simulink model "top_model_rw_desatTest"  (R2017b)
settings: Solver=FixedStepAuto  StartTime=0.0  StopTime=30000  FixedStep=.2  RelTol=1e-3  EnableMultiTasking=on
model workspace: external: MATLAB File C:\Users\Justin\Documents\00 MEng Project\PAN_ADCS\initialization\simulink_workspace_init.m (data not in the file)
undefined symbols (not defined in the file): h_init, hdmax, hmax, IAU, Imp_max, Imp_min, init, K_F, Kd, km, Kp, L_F, m_follower, match_tol, muE, ontime_max, ontime_min, q_init, s, Thrust_max, Thrust_min, wbn_init
libraries: aerolibtransform2 x12, aerolibconvert2 x8, sharedtransform x8, hEemethod x8, aerolibgravity2 x6, aerolibutil x6, aerolibcelestial x4, vrlib x4
(part 1 of 5)
settings Model: Creator=The MathWorks, Inc.  LastModifiedBy=Justin
settings DataIOCC: LimitDataPoints=on
settings OptimizationCC: LifeSpan=inf
settings DebuggingCC: AllowSymbolicDim=off  SFUnexpectedBacktrackingDiag=warning  SFNoUnconditionalDefaultTransitionDiag=warning  SFExecutionAtInitializationDiag=none
settings ModelReferenceCC: PropagateSignalLabelsOutOfModel=off
settings CodeAppCC: StateflowObjectComments=on
settings GRTTargetCC: TargetLangStandard=C89/C90 (ANSI)
settings ConfigComp: CovMetricSettings=dw  CovHtmlReporting=on  CovSaveCumulativeToWorkspaceVar=on  CovSaveSingleToWorkspaceVar=on  CovExternalEMLEnable=off

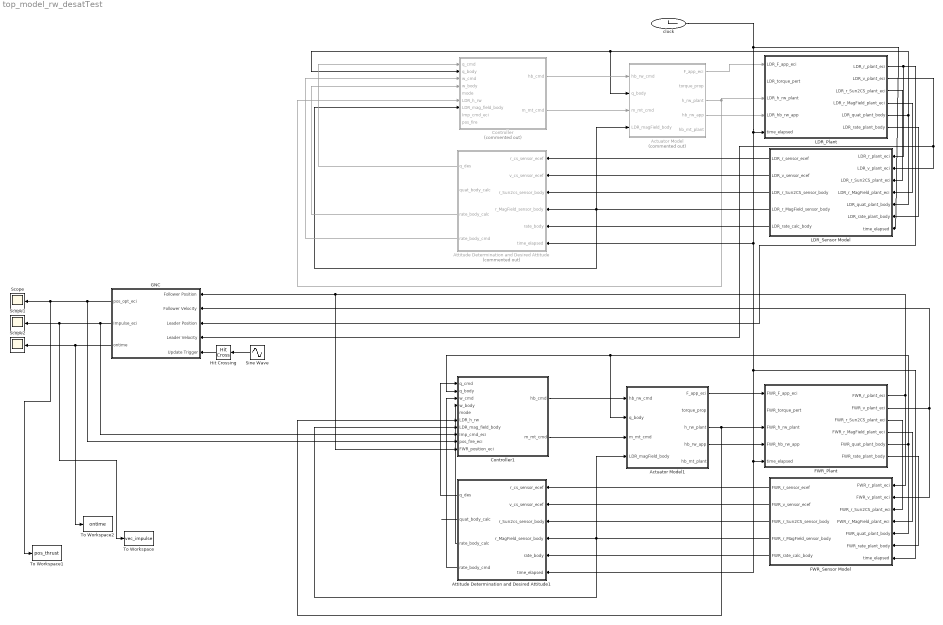
== system top_model_rw_desatTest ==
  Actuator Model : Subsystem  Commented=on
  Actuator Model1 : Subsystem
  Attitude Determination and Desired Attitude : Subsystem  Commented=on
  Attitude Determination and Desired Attitude1 : Subsystem
  Controller : Subsystem  Commented=on
  Controller1 : Subsystem
  FWR_Plant : Subsystem
  FWR_Sensor Model : Subsystem
  GNC : Subsystem
  Hit Crossing : HitCross  HitCrossingOffset=0.5  HitCrossingDirection=rising
  LDR_Plant : Subsystem
  LDR_Sensor Model : Subsystem
  Scope : Scope
  Scope1 : Scope
  Scope2 : Scope
  Sine Wave : Sin  Frequency=2*pi/550  SampleTime=0
  To Workspace : ToWorkspace  VariableName=vec_impulse  SaveFormat=Timeseries  SampleTime=-1
  To Workspace1 : ToWorkspace  VariableName=pos_thrust  SaveFormat=Timeseries  SampleTime=-1
  To Workspace2 : ToWorkspace  VariableName=ontime  SaveFormat=Timeseries  SampleTime=-1
  clock : Clock
      settings: Decimation=100
  wires:
  LDR_Plant/3(LDR_r_Sun2CS_plant_eci) -> LDR_Sensor Model/3(LDR_r_Sun2CS_plant_eci)
  LDR_Plant/4(LDR_r_MagField_plant_eci) -> LDR_Sensor Model/4(LDR_r_MagField_plant_eci)
  LDR_Plant/6(LDR_rate_plant_body) -> LDR_Sensor Model/6(LDR_rate_plant_body)
  Actuator Model/1(F_app_eci) -> LDR_Plant/1(LDR_F_app_eci)
  Actuator Model/3(h_rw_plant) -> Controller/6(LDR_h_rw), LDR_Plant/3(LDR_h_rw_plant)
  Actuator Model/4(hb_rw_app) -> LDR_Plant/4(LDR_hb_rw_app)
  LDR_Sensor Model/1(LDR_r_sensor_ecef) -> Attitude Determination and Desired Attitude/1(r_cs_sensor_ecef)
  LDR_Sensor Model/2(LDR_v_sensor_ecef) -> Attitude Determination and Desired Attitude/2(v_cs_sensor_ecef)
  LDR_Sensor Model/3(LDR_r_Sun2CS_sensor_body) -> Attitude Determination and Desired Attitude/3(r_Sun2cs_sensor_body)
  LDR_Sensor Model/4(LDR_r_MagField_sensor_body) -> Controller/7(LDR_mag_field_body), Attitude Determination and Desired Attitude/4(r_MagField_sensor_body), Actuator Model/4(LDR_magField_body)
  LDR_Sensor Model/5(LDR_rate_calc_body) -> Attitude Determination and Desired Attitude/5(rate_body)
  GNC/1(pos_opt_eci) -> Controller1/9(pos_fire_eci), To Workspace1/1, Scope/1
  GNC/2(Impulse_eci) -> Controller1/8(Imp_cmd_eci), To Workspace/1, Scope1/1
  GNC/3(ontime) -> To Workspace2/1, Scope2/1
  Sine Wave/1 -> Hit Crossing/1
  Hit Crossing/1 -> GNC/5(Update Trigger)
  LDR_Plant/5(LDR_quat_plant_body) -> LDR_Sensor Model/5(LDR_quat_plant_body), Actuator Model/2(q_body), Controller/2(q_body)
  Attitude Determination and Desired Attitude/1(q_des) -> Controller/1(q_cmd)
  Attitude Determination and Desired Attitude/3(rate_body_calc) -> Controller/4(w_body)
  Controller/1(hb_cmd) -> Actuator Model/1(hb_rw_cmd)
  Controller/2(m_mt_cmd) -> Actuator Model/3(m_mt_cmd)
  Attitude Determination and Desired Attitude/4(rate_body_cmd) -> Controller/3(w_cmd)
  LDR_Plant/1(LDR_r_plant_eci) -> GNC/3(Leader Position), LDR_Sensor Model/1(LDR_r_plant_eci)
  LDR_Plant/2(LDR_v_plant_eci) -> GNC/4(Leader Velocity), LDR_Sensor Model/2(LDR_v_plant_eci)
  FWR_Plant/2(FWR_v_plant_eci) -> FWR_Sensor Model/2(FWR_v_plant_eci), GNC/2(Follower Velocity)
  FWR_Plant/5(FWR_quat_plant_body) -> FWR_Sensor Model/5(FWR_quat_plant_body), Actuator Model1/2(q_body), Controller1/2(q_body)
  Controller1/2(m_mt_cmd) -> Actuator Model1/3(m_mt_cmd)
  FWR_Sensor Model/3(FWR_r_Sun2CS_sensor_body) -> Attitude Determination and Desired Attitude1/3(r_Sun2cs_sensor_body)
  FWR_Sensor Model/2(FWR_v_sensor_ecef) -> Attitude Determination and Desired Attitude1/2(v_cs_sensor_ecef)
  FWR_Sensor Model/1(FWR_r_sensor_ecef) -> Attitude Determination and Desired Attitude1/1(r_cs_sensor_ecef)
  Controller1/1(hb_cmd) -> Actuator Model1/1(hb_rw_cmd)
  FWR_Plant/3(FWR_r_Sun2CS_plant_eci) -> FWR_Sensor Model/3(FWR_r_Sun2CS_plant_eci)
  FWR_Plant/6(FWR_rate_plant_body) -> FWR_Sensor Model/6(FWR_rate_plant_body)
  FWR_Sensor Model/4(FWR_r_MagField_sensor_body) -> Controller1/7(LDR_mag_field_body), Attitude Determination and Desired Attitude1/4(r_MagField_sensor_body), Actuator Model1/4(LDR_magField_body)
  Actuator Model1/3(h_rw_plant) -> Controller1/6(LDR_h_rw), FWR_Plant/3(FWR_h_rw_plant)
  clock/1 -> LDR_Sensor Model/7(time_elapsed), FWR_Sensor Model/7(time_elapsed), Attitude Determination and Desired Attitude1/6(time_elapsed), FWR_Plant/5(time_elapsed), Attitude Determination and Desired Attitude/6(time_elapsed), LDR_Plant/5(time_elapsed)
  Actuator Model1/4(hb_rw_app) -> FWR_Plant/4(FWR_hb_rw_app)
  FWR_Plant/4(FWR_r_MagField_plant_eci) -> FWR_Sensor Model/4(FWR_r_MagField_plant_eci)
  FWR_Sensor Model/5(FWR_rate_calc_body) -> Attitude Determination and Desired Attitude1/5(rate_body)
  Attitude Determination and Desired Attitude1/1(q_des) -> Controller1/1(q_cmd)
  Attitude Determination and Desired Attitude1/2(quat_body_calc) -> ?
  Attitude Determination and Desired Attitude1/3(rate_body_calc) -> Controller1/4(w_body)
  Attitude Determination and Desired Attitude1/4(rate_body_cmd) -> Controller1/3(w_cmd)
  Actuator Model1/1(F_app_eci) -> FWR_Plant/1(FWR_F_app_eci)
  FWR_Plant/1(FWR_r_plant_eci) -> Controller1/10(FWR_position_eci), GNC/1(Follower Position), FWR_Sensor Model/1(FWR_r_plant_eci)

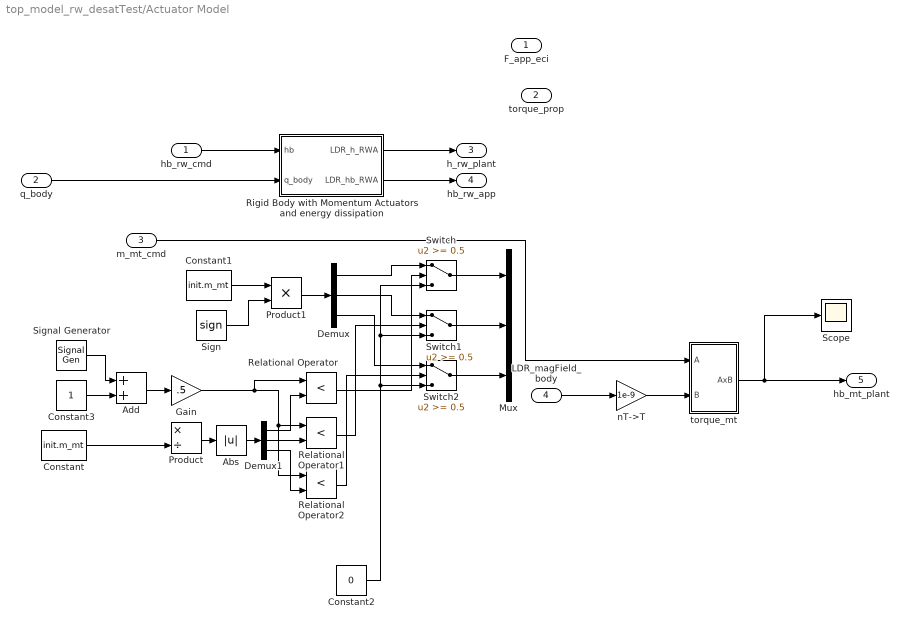
== system top_model_rw_desatTest/Actuator Model ==
  hb_rw_cmd : Inport
  q_body : Inport  Port=2
  m_mt_cmd : Inport  Port=3
  LDR_magField_body : Inport  Port=4
  Abs : Abs  SaturateOnIntegerOverflow=on
  Add : Sum
  Constant : Constant  Value=init.m_mt
  Constant1 : Constant  Value=init.m_mt
  Constant2 : Constant  Value=0
  Constant3 : Constant
  Demux : Demux  Outputs=3
  Demux1 : Demux  Outputs=3
  Gain : Gain  Gain=.5
  Mux : Mux  Inputs=3
  Product : Product  Inputs=*/
  Product1 : Product
  Relational Operator : RelationalOperator  Operator=<  OutDataTypeStr=boolean  RndMeth=Simplest
  Relational Operator1 : RelationalOperator  Operator=<  OutDataTypeStr=boolean  RndMeth=Simplest
  Relational Operator2 : RelationalOperator  Operator=<  OutDataTypeStr=boolean  RndMeth=Simplest
  Rigid Body with Momentum Actuators and energy dissipation : Subsystem
  Scope : Scope
  Sign : Signum
  Signal Generator : SignalGenerator  WaveForm=sawtooth  Frequency=.5
  Switch : Switch  Threshold=0.5  SaturateOnIntegerOverflow=on  InputSameDT=on
  Switch1 : Switch  Threshold=0.5  SaturateOnIntegerOverflow=on  InputSameDT=on
  Switch2 : Switch  Threshold=0.5  SaturateOnIntegerOverflow=on  InputSameDT=on
  nT->T : Gain  Gain=1e-9
  torque_mt : Subsystem
  F_app_eci : Outport
  torque_prop : Outport  Port=2
  h_rw_plant : Outport  Port=3
  hb_rw_app : Outport  Port=4
  hb_mt_plant : Outport  Port=5
  wires:
  Rigid Body with Momentum Actuators and energy dissipation/1(LDR_h_RWA) -> h_rw_plant/1
  Rigid Body with Momentum Actuators and energy dissipation/2(LDR_hb_RWA) -> hb_rw_app/1
  hb_rw_cmd/1 -> Rigid Body with Momentum Actuators and energy dissipation/1(hb)
  q_body/1 -> Rigid Body with Momentum Actuators and energy dissipation/2(q_body)
  LDR_magField_body/1 -> nT->T/1
  nT->T/1 -> torque_mt/2(B)
  torque_mt/1(AxB) -> hb_mt_plant/1, Scope/1
  Constant/1 -> Product/2
  Product/1 -> Abs/1
  Constant1/1 -> Product1/1
  Sign/1 -> Product1/2
  Product1/1 -> Demux/1
  Switch2/1 -> Mux/3
  Switch1/1 -> Mux/2
  Switch/1 -> Mux/1
  Demux/1 -> Switch/1
  Demux/2 -> Switch1/1
  Demux/3 -> Switch2/1
  Relational Operator/1 -> Switch/2
  Relational Operator1/1 -> Switch1/2
  Relational Operator2/1 -> Switch2/2
  Constant2/1 -> Switch/3, Switch1/3, Switch2/3
  Abs/1 -> Demux1/1
  Demux1/1 -> Relational Operator/2
  Demux1/2 -> Relational Operator1/2
  Demux1/3 -> Relational Operator2/2
  Signal Generator/1 -> Add/1
  Constant3/1 -> Add/2
  Add/1 -> Gain/1
  Gain/1 -> Relational Operator2/1, Relational Operator1/1, Relational Operator/1
  m_mt_cmd/1 -> torque_mt/1(A)

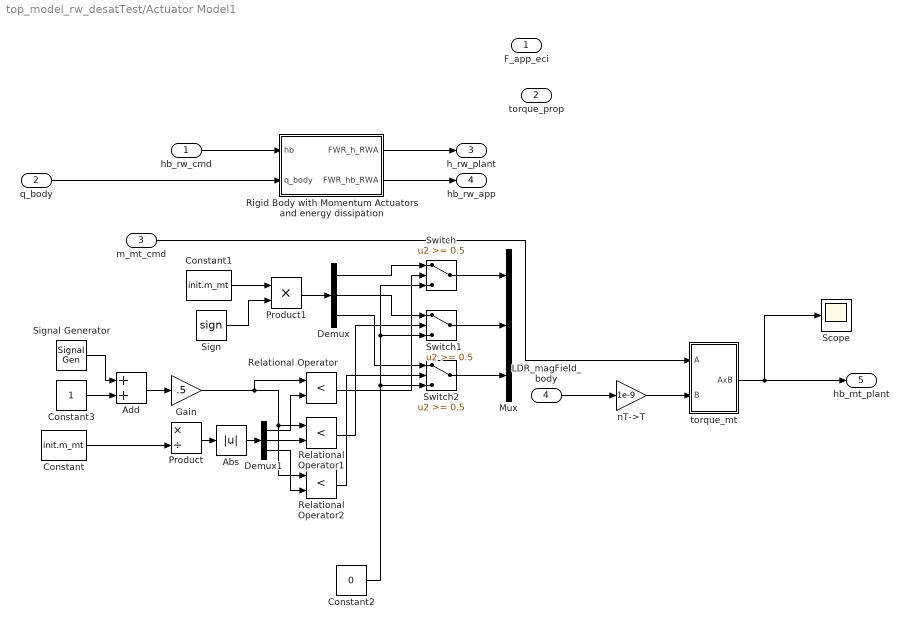
== system top_model_rw_desatTest/Actuator Model1 ==
  hb_rw_cmd : Inport
  q_body : Inport  Port=2
  m_mt_cmd : Inport  Port=3
  LDR_magField_body : Inport  Port=4
  Abs : Abs  SaturateOnIntegerOverflow=on
  Add : Sum
  Constant : Constant  Value=init.m_mt
  Constant1 : Constant  Value=init.m_mt
  Constant2 : Constant  Value=0
  Constant3 : Constant
  Demux : Demux  Outputs=3
  Demux1 : Demux  Outputs=3
  Gain : Gain  Gain=.5
  Mux : Mux  Inputs=3
  Product : Product  Inputs=*/
  Product1 : Product
  Relational Operator : RelationalOperator  Operator=<  OutDataTypeStr=boolean  RndMeth=Simplest
  Relational Operator1 : RelationalOperator  Operator=<  OutDataTypeStr=boolean  RndMeth=Simplest
  Relational Operator2 : RelationalOperator  Operator=<  OutDataTypeStr=boolean  RndMeth=Simplest
  Rigid Body with Momentum Actuators and energy dissipation : Subsystem
  Scope : Scope
  Sign : Signum
  Signal Generator : SignalGenerator  WaveForm=sawtooth  Frequency=.5
  Switch : Switch  Threshold=0.5  SaturateOnIntegerOverflow=on  InputSameDT=on
  Switch1 : Switch  Threshold=0.5  SaturateOnIntegerOverflow=on  InputSameDT=on
  Switch2 : Switch  Threshold=0.5  SaturateOnIntegerOverflow=on  InputSameDT=on
  nT->T : Gain  Gain=1e-9
  torque_mt : Subsystem
  F_app_eci : Outport
  torque_prop : Outport  Port=2
  h_rw_plant : Outport  Port=3
  hb_rw_app : Outport  Port=4
  hb_mt_plant : Outport  Port=5
  wires:
  Rigid Body with Momentum Actuators and energy dissipation/1(FWR_h_RWA) -> h_rw_plant/1
  Rigid Body with Momentum Actuators and energy dissipation/2(FWR_hb_RWA) -> hb_rw_app/1
  hb_rw_cmd/1 -> Rigid Body with Momentum Actuators and energy dissipation/1(hb)
  q_body/1 -> Rigid Body with Momentum Actuators and energy dissipation/2(q_body)
  LDR_magField_body/1 -> nT->T/1
  nT->T/1 -> torque_mt/2(B)
  torque_mt/1(AxB) -> hb_mt_plant/1, Scope/1
  Constant/1 -> Product/2
  Product/1 -> Abs/1
  Constant1/1 -> Product1/1
  Sign/1 -> Product1/2
  Product1/1 -> Demux/1
  Switch2/1 -> Mux/3
  Switch1/1 -> Mux/2
  Switch/1 -> Mux/1
  Demux/1 -> Switch/1
  Demux/2 -> Switch1/1
  Demux/3 -> Switch2/1
  Relational Operator/1 -> Switch/2
  Relational Operator1/1 -> Switch1/2
  Relational Operator2/1 -> Switch2/2
  Constant2/1 -> Switch/3, Switch1/3, Switch2/3
  Abs/1 -> Demux1/1
  Demux1/1 -> Relational Operator/2
  Demux1/2 -> Relational Operator1/2
  Demux1/3 -> Relational Operator2/2
  Signal Generator/1 -> Add/1
  Constant3/1 -> Add/2
  Add/1 -> Gain/1
  Gain/1 -> Relational Operator2/1, Relational Operator1/1, Relational Operator/1
  m_mt_cmd/1 -> torque_mt/1(A)

== system top_model_rw_desatTest/Attitude Determination and Desired Attitude ==
  r_cs_sensor_ecef : Inport
  v_cs_sensor_ecef : Inport  Port=2
  r_Sun2cs_sensor_body : Inport  Port=3
  r_MagField_sensor_body : Inport  Port=4
  rate_body : Inport  Port=5
  time_elapsed : Inport  Port=6
  Attitude Determination : Subsystem
  Cross3 : Subsystem
  Demux1 : Demux
  Demux2 : Demux
  Direction Cosine Matrix to Quaternions : sharedtransform/Direction Cosine Matrix  to Quaternions  Commented=on
      settings: SourceProductName=Aerospace Blockset  SourceProductBaseCode=AE
  ECEF2ECI : Subsystem
  ECEF2ECI1 : Subsystem
  Position and Velocity to Desired Attitude in Quat : Subsystem
  Product : Product  Inputs=/*
  Product1 : Product
  Quaternions to Direction Cosine Matrix : sharedtransform/Quaternions to  Direction Cosine Matrix  Commented=on
      settings: SourceProductName=Aerospace Blockset  SourceProductBaseCode=AE
  Quaternions to Rotation Angles : sharedtransform/Quaternions to Rotation Angles  Commented=on  rotationOrder=ZYX
      settings: SourceProductBaseCode=AE
  Rotation Angles to Direction Cosine Matrix : sharedtransform/Rotation Angles to Direction Cosine Matrix  Commented=on  rotationOrder=ZYX
      settings: SourceProductBaseCode=AE
  norm : Subsystem
  norm1 : Subsystem
  normalize : Subsystem
  q_calc : Scope  NumInputPorts=4
  q_ref : Scope  NumInputPorts=4
  q_des : Outport
  quat_body_calc : Outport  Port=2
  rate_body_calc : Outport  Port=3
  rate_body_cmd : Outport  Port=4
  wires:
  rate_body/1 -> rate_body_calc/1
  time_elapsed/1 -> ECEF2ECI1/2(sec), ECEF2ECI/2(sec), Attitude Determination/1(time_elapsed)
  r_cs_sensor_ecef/1 -> ECEF2ECI/1(ecef)
  v_cs_sensor_ecef/1 -> ECEF2ECI1/1(ecef)
  ECEF2ECI/1(eci) -> norm/1(v), Cross3/2(B), Attitude Determination/2(r_cs_sensor_eci), Position and Velocity to Desired Attitude in Quat/1(r_cs_sensor_eci)
  ECEF2ECI1/1(eci) -> norm1/1(v), Cross3/1(A), Position and Velocity to Desired Attitude in Quat/2(v_cs_sensor_eci)
  r_Sun2cs_sensor_body/1 -> Attitude Determination/3(r_Sun2cs_sensor_body)
  r_MagField_sensor_body/1 -> Attitude Determination/4(r_MagField_sensor_body)
  Attitude Determination/1(quat_body_calc) -> Demux1/1, quat_body_calc/1
  Demux1/2 -> q_calc/2
  Demux1/1 -> q_calc/1
  Demux1/3 -> q_calc/3
  Demux1/4 -> q_calc/4
  Position and Velocity to Desired Attitude in Quat/1(q_des) -> Demux2/1, q_des/1
  Demux2/2 -> q_ref/2
  Demux2/1 -> q_ref/1
  Demux2/3 -> q_ref/3
  Demux2/4 -> q_ref/4
  Cross3/1(AxB) -> normalize/1(v)
  norm/1(|v|) -> Product/1
  norm1/1(|v|) -> Product/2
  Product/1 -> Product1/2
  normalize/1(v_hat) -> Product1/1
  Product1/1 -> rate_body_cmd/1

== system top_model_rw_desatTest/Attitude Determination and Desired Attitude1 ==
  r_cs_sensor_ecef : Inport
  v_cs_sensor_ecef : Inport  Port=2
  r_Sun2cs_sensor_body : Inport  Port=3
  r_MagField_sensor_body : Inport  Port=4
  rate_body : Inport  Port=5
  time_elapsed : Inport  Port=6
  Attitude Determination : Subsystem
  Cross3 : Subsystem
  Demux1 : Demux
  Demux2 : Demux
  Demux3 : Demux  Outputs=3
  Direction Cosine Matrix to Quaternions : sharedtransform/Direction Cosine Matrix  to Quaternions  Commented=on
      settings: SourceProductName=Aerospace Blockset  SourceProductBaseCode=AE
  ECEF2ECI : Subsystem
  ECEF2ECI1 : Subsystem
  Position and Velocity to Desired Attitude in Quat : Subsystem
  Product : Product  Inputs=/*
  Product1 : Product
  Quaternions to Direction Cosine Matrix : sharedtransform/Quaternions to  Direction Cosine Matrix  Commented=on
      settings: SourceProductName=Aerospace Blockset  SourceProductBaseCode=AE
  Quaternions to Rotation Angles : sharedtransform/Quaternions to Rotation Angles  Commented=on  rotationOrder=ZYX
      settings: SourceProductBaseCode=AE
  Rotation Angles to Direction Cosine Matrix : sharedtransform/Rotation Angles to Direction Cosine Matrix  Commented=on  rotationOrder=ZYX
      settings: SourceProductBaseCode=AE
  norm : Subsystem
  norm1 : Subsystem
  normalize : Subsystem
  q_calc : Scope  NumInputPorts=4
  q_ref : Scope  NumInputPorts=4
  wbn_cmd : Scope  NumInputPorts=3
  q_des : Outport
  quat_body_calc : Outport  Port=2
  rate_body_calc : Outport  Port=3
  rate_body_cmd : Outport  Port=4
  wires:
  rate_body/1 -> rate_body_calc/1
  time_elapsed/1 -> ECEF2ECI1/2(sec), ECEF2ECI/2(sec), Attitude Determination/1(time_elapsed)
  r_cs_sensor_ecef/1 -> ECEF2ECI/1(ecef)
  v_cs_sensor_ecef/1 -> ECEF2ECI1/1(ecef)
  ECEF2ECI/1(eci) -> norm/1(v), Cross3/2(B), Attitude Determination/2(r_cs_sensor_eci), Position and Velocity to Desired Attitude in Quat/1(r_cs_sensor_eci)
  ECEF2ECI1/1(eci) -> norm1/1(v), Cross3/1(A), Position and Velocity to Desired Attitude in Quat/2(v_cs_sensor_eci)
  r_Sun2cs_sensor_body/1 -> Attitude Determination/3(r_Sun2cs_sensor_body)
  r_MagField_sensor_body/1 -> Attitude Determination/4(r_MagField_sensor_body)
  Attitude Determination/1(quat_body_calc) -> Demux1/1, quat_body_calc/1
  Demux1/2 -> q_calc/2
  Demux1/1 -> q_calc/1
  Demux1/3 -> q_calc/3
  Demux1/4 -> q_calc/4
  Position and Velocity to Desired Attitude in Quat/1(q_des) -> Demux2/1, q_des/1
  Demux2/2 -> q_ref/2
  Demux2/1 -> q_ref/1
  Demux2/3 -> q_ref/3
  Demux2/4 -> q_ref/4
  Cross3/1(AxB) -> normalize/1(v)
  norm/1(|v|) -> Product/1
  norm1/1(|v|) -> Product/2
  Product/1 -> Product1/2
  normalize/1(v_hat) -> Product1/1
  Demux3/1 -> wbn_cmd/1
  Product1/1 -> Demux3/1, rate_body_cmd/1
  Demux3/3 -> wbn_cmd/3
  Demux3/2 -> wbn_cmd/2

== system top_model_rw_desatTest/Controller ==
  note: 0- Power ON / Restart
      | 1- Detumble
      | 2- Regulation Control
      | 3- Tracking Control
      | 4- Thermal Safe
      | 5- Power Max
      | 6- Large Angle Slew
  note: 0- Power ON/restart
      | 1- Safe hold
      | 2- Detumble
      | 3- Large angle slew
      | 4- Normal
      | 5- Eclipse
      | 6- Docking
  q_cmd : Inport
  q_body : Inport  Port=2
  w_cmd : Inport  Port=3
  w_body : Inport  Port=4
  mode : Inport  Port=5
  LDR_h_rw : Inport  Port=6
  LDR_mag_field_body : Inport  Port=7
  Imp_cmd_eci : Inport  Port=8
  pos_fire : Inport  Port=9
  Free Rigid Body with Momentum Actuators2 : Subsystem  Commented=on
  If : If  IfExpression=u1 == 0  ElseIfExpressions=u1 == 1, u1 == 2, u1 == 3, u1 == 4, u1==5
  Impulse_eci2body : Product  Commented=on  Multiplication=Matrix(*)
  Mode Generator : Stateflow chart  Commented=on  TreatAsAtomicUnit=on
  Normal Mode Control System : Subsystem  TreatAsAtomicUnit=on
  Propulsion : Subsystem  Commented=on
  TestNormalMode : Constant  Value=4
  quat to DCM : Subsystem  Commented=on  mask(Direction Cosine Matrix){}
      mask help: Determines the 3x3 Direction Cosine Matrix (DCM) from a 4x1 quaternion orientation vector. The outputted DCM transforms vectors from inertial axes to body axes. This version corrects the fucked-up MATLAB one.
      mask Help:
      | <p>This block determines the 3x3 Direction Cosine Matrix (DCM) from a 4x1 quaternion orientation vector. The outputted DCM transforms vectors from inertial axes to body axes.  This version corrects the fucked-up MATLAB one</p>
      | 
      | <p>The block input and output contain more than one signal as described below.</p>
      | 
      | <p><H4>Block Vector Input - Quaternion</H4>
      | <ul>
      | <li>q0</li>
      | <li>q1</li>
      | <li>q2</li>
      | <li>q3</li>
      | </ul>
      | </p>
      | 
      | <p><H4>Block Matrix Output - Direction Cosine Matrix  </H4>
      |     <ul>
      |    </ul>
      |    </p>
      mask Display: disp('q to Q')
  hb_cmd : Outport
  m_mt_cmd : Outport  Port=2
  wires:
  q_cmd/1 -> Normal Mode Control System/1(q_cmd)
  q_body/1 -> quat to DCM/1(e0 e1 e2 e3), Normal Mode Control System/2(q_body)
  w_cmd/1 -> Normal Mode Control System/3(w_cmd)
  w_body/1 -> Normal Mode Control System/4(w_body)
  TestNormalMode/1 -> If/1
  If/5 -> Normal Mode Control System/Action
  Normal Mode Control System/1(hb_rw_cmd) -> hb_cmd/1
  LDR_mag_field_body/1 -> Normal Mode Control System/6(LDR_mag_field_body)
  Normal Mode Control System/2(m_mt_cmd) -> m_mt_cmd/1
  LDR_h_rw/1 -> Normal Mode Control System/5(LDR_h_rw)
  Imp_cmd_eci/1 -> Impulse_eci2body/2
  Impulse_eci2body/1 -> Propulsion/1(Impulse_cmd_body)
  quat to DCM/1(DCM) -> Impulse_eci2body/1
  pos_fire/1 -> Propulsion/2(pos_fire)
  Propulsion/1(Force_applied) -> ?

== system top_model_rw_desatTest/Controller1 ==
  note: 0- Power ON / Restart
      | 1- Detumble
      | 2- Regulation Control
      | 3- Tracking Control
      | 4- Thermal Safe
      | 5- Power Max
      | 6- Large Angle Slew
  note: 0- Power ON/restart
      | 1- Safe hold
      | 2- Detumble
      | 3- Large angle slew
      | 4- Normal
      | 5- Eclipse
      | 6- Docking
  q_cmd : Inport
  q_body : Inport  Port=2
  w_cmd : Inport  Port=3
  w_body : Inport  Port=4
  mode : Inport  Port=5
  LDR_h_rw : Inport  Port=6
  LDR_mag_field_body : Inport  Port=7
  Imp_cmd_eci : Inport  Port=8
  pos_fire_eci : Inport  Port=9
  FWR_position_eci : Inport  Port=10
  Constant : Constant  Value=1000
  Free Rigid Body with Momentum Actuators2 : Subsystem  Commented=on
  Hit Crossing1 : HitCross  HitCrossingDirection=falling
  If : If  IfExpression=u1 == 0  ElseIfExpressions=u1 == 1, u1 == 2, u1 == 3, u1 == 4, u1==5
  Impulse_eci2body : Product  Multiplication=Matrix(*)
  Mode Generator : Stateflow chart  Commented=on  TreatAsAtomicUnit=on
  Normal Mode Control System : Subsystem  TreatAsAtomicUnit=on
  Propulsion : Subsystem
  Scope : Scope
  Scope1 : Scope
  Sum : Sum  Inputs=|+-
  Sum2 : Sum  Inputs=|+-
  TestNormalMode : Constant  Value=4
  norm : Subsystem
  quat to DCM : Subsystem  mask(Direction Cosine Matrix){}
      mask help: Determines the 3x3 Direction Cosine Matrix (DCM) from a 4x1 quaternion orientation vector. The outputted DCM transforms vectors from inertial axes to body axes. This version corrects the fucked-up MATLAB one.
      mask Help:
      | <p>This block determines the 3x3 Direction Cosine Matrix (DCM) from a 4x1 quaternion orientation vector. The outputted DCM transforms vectors from inertial axes to body axes.  This version corrects the fucked-up MATLAB one</p>
      | 
      | <p>The block input and output contain more than one signal as described below.</p>
      | 
      | <p><H4>Block Vector Input - Quaternion</H4>
      | <ul>
      | <li>q0</li>
      | <li>q1</li>
      | <li>q2</li>
      | <li>q3</li>
      | </ul>
      | </p>
      | 
      | <p><H4>Block Matrix Output - Direction Cosine Matrix  </H4>
      |     <ul>
      |    </ul>
      |    </p>
      mask Display: disp('q to Q')
  hb_cmd : Outport
  m_mt_cmd : Outport  Port=2
  wires:
  q_cmd/1 -> Normal Mode Control System/1(q_cmd)
  q_body/1 -> quat to DCM/1(e0 e1 e2 e3), Normal Mode Control System/2(q_body)
  w_cmd/1 -> Normal Mode Control System/3(w_cmd)
  w_body/1 -> Normal Mode Control System/4(w_body)
  TestNormalMode/1 -> If/1
  If/5 -> Normal Mode Control System/Action
  Normal Mode Control System/1(hb_rw_cmd) -> hb_cmd/1
  LDR_mag_field_body/1 -> Normal Mode Control System/6(LDR_mag_field_body)
  Normal Mode Control System/2(m_mt_cmd) -> m_mt_cmd/1
  LDR_h_rw/1 -> Normal Mode Control System/5(LDR_h_rw)
  Imp_cmd_eci/1 -> Impulse_eci2body/2
  Impulse_eci2body/1 -> Propulsion/1(Impulse_cmd_body)
  quat to DCM/1(DCM) -> Impulse_eci2body/1
  pos_fire_eci/1 -> Sum/1
  Propulsion/1(Force_applied) -> ?
  FWR_position_eci/1 -> Sum/2
  Sum/1 -> norm/1(v)
  norm/1(|v|) -> Scope1/1, Sum2/1
  Constant/1 -> Sum2/2
  Sum2/1 -> Hit Crossing1/1
  Hit Crossing1/1 -> Propulsion/2(trigger), Scope/1

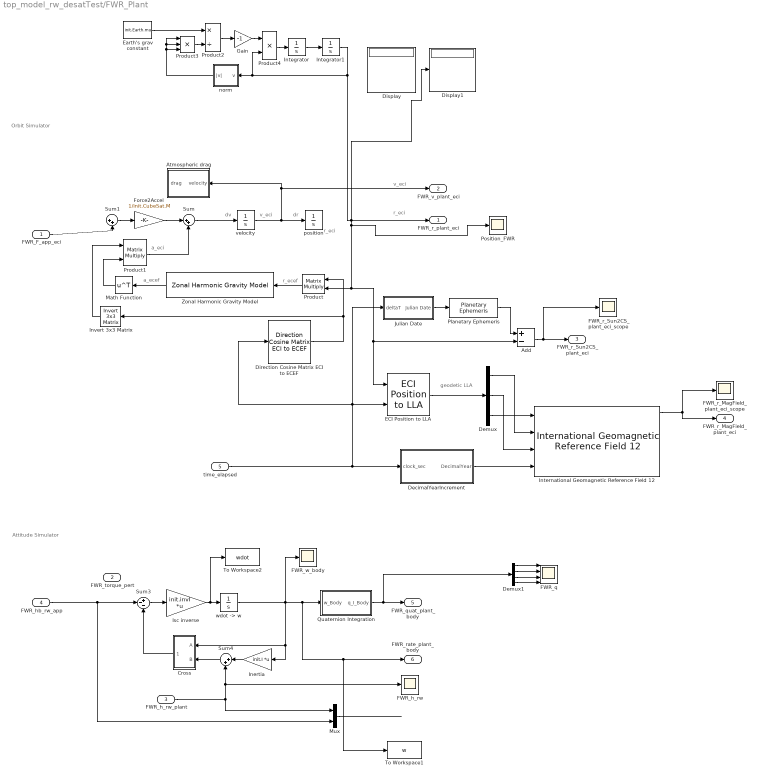
== system top_model_rw_desatTest/FWR_Plant ==
  note: a_ecef
  note: v_eci
  note: a_eci
  note: geodetic LLA
  note: r_ecef
  note: Orbit Simulator
  note: v_eci
  note: dv
  note: r_eci
  note: r_eci
  note: dr
  note: Attitude Simulator
  FWR_F_app_eci : Inport
  "FWR_torque_pert " : Inport  Port=2
  FWR_h_rw_plant : Inport  Port=3
  FWR_hb_rw_app : Inport  Port=4
  time_elapsed : Inport  Port=5
  Add : Sum  Inputs=+-
  Atmospheric drag : MATLAB Function  TreatAsAtomicUnit=on
  Cross : Subsystem
  DecimalYearIncrement : Subsystem
  Demux : Demux  Outputs=3
  Demux1 : Demux
  Direction Cosine Matrix ECI to ECEF : aerolibtransform2/Direction Cosine Matrix ECI to ECEF  red=IAU-2000/2006  year=init.year  month=October  day=20  hour=init.hour  min=init.min  sec=init.sec  deltaT=Sec  errorflag=Error  extraparamflag=off
      settings: AttributesFormatString=%<red>  SourceProductName=Aerospace Blockset  SourceProductBaseCode=AE
  Display : Display
  Display1 : Display
  ECI Position to LLA : aerolibtransform2/ECI Position to LLA  red=IAU-2000/2006  year=init.year  month=October  day=20  hour=init.hour  min=init.min  sec=init.sec  deltaT=Sec  errorflag=Error  extraparamflag=off  eunits=Metric (MKS)  earthmodel=WGS84  flat=1/298.257223563  eqradius=6378137
      settings: AttributesFormatString=%<red>  SourceProductName=Aerospace Blockset  SourceProductBaseCode=AE
  Earth's grav constant : Constant  Value=init.Earth.mu
  "FWR_h_rw " : Scope
  FWR_q : Scope  NumInputPorts=4
  FWR_r_MagField_plant_eci_scope : Scope
  FWR_r_Sun2CS_plant_eci_scope : Scope
  FWR_w_body : Scope
  Force2Accel : Gain  Gain=1/init.CubeSat.M
  Gain : Gain  Gain=-1  SaturateOnIntegerOverflow=on  OutDataTypeStr=Inherit: Same as input  ParamDataTypeStr=Inherit: Same as input
  Inertia : Gain  Gain=init.I  Multiplication=Matrix(K*u)  SaturateOnIntegerOverflow=on  OutDataTypeStr=Inherit: Same as input  ParamDataTypeStr=Inherit: Same as input
  Integrator : Integrator  InitialCondition=init.FWR.V
  Integrator1 : Integrator  InitialCondition=init.FWR.P
  International Geomagnetic Reference Field 12 : aerolibgravity2/International Geomagnetic Reference Field 12  units=Metric (MKS)  time_in=on  month=January  day=1  year=2020  action=None  sv_out=off
      settings: SourceProductName=Aerospace Blockset  SourceProductBaseCode=AE
  Invert 3x3 Matrix : aerolibutil/Invert  3x3 Matrix
  Isc inverse : Gain  Gain=init.invI  Multiplication=Matrix(K*u)  SaturateOnIntegerOverflow=on  OutDataTypeStr=Inherit: Same as input  ParamDataTypeStr=Inherit: Same as input
  Julian Date : Subsystem
  Math Function : Math  Operator=transpose  SaturateOnIntegerOverflow=on
  Mux : Mux  Inputs=2
  Planetary Ephemeris : aerolibcelestial/Planetary Ephemeris  kmflag=km,km/s  epochflag=Julian date  de=DE430  nCenter=Earth  nTarget=Sun  errorflag=Error  velflag=off
      settings: SourceProductName=Aerospace Blockset  SourceProductBaseCode=AE
  Position_FWR : Scope
  Product : Product  Multiplication=Matrix(*)
  Product1 : Product  Multiplication=Matrix(*)
  Product2 : Product  Inputs=*/  SaturateOnIntegerOverflow=on  OutDataTypeStr=Inherit: Same as first input
  Product3 : Product  Inputs=***  SaturateOnIntegerOverflow=on  OutDataTypeStr=Inherit: Same as first input
  Product4 : Product  Inputs=**  SaturateOnIntegerOverflow=on  OutDataTypeStr=Inherit: Same as first input
  Quaternion Integration : Subsystem
  Sum : Sum  Inputs=|++
  Sum1 : Sum  Inputs=|++
  Sum3 : Sum  Inputs=+--  SaturateOnIntegerOverflow=on  InputSameDT=on  OutDataTypeStr=Inherit: Same as first input
  Sum4 : Sum  Inputs=|++
  To Workspace1 : ToWorkspace  VariableName=w  SaveFormat=Timeseries  SampleTime=-1
  To Workspace2 : ToWorkspace  VariableName=wdot  SaveFormat=Timeseries  SampleTime=-1
  Zonal Harmonic Gravity Model : aerolibgravity2/Zonal Harmonic Gravity Model  units=Metric (MKS)  degree=4  action=Warning  ptype=Earth  R=6378136.3  GM=398600441500000  jvalue=[1.0826269e-03 -2.5323000e-06 -1.6204000e-06]
      settings: SourceProductName=Aerospace Blockset  SourceProductBaseCode=AE
  norm : Subsystem
  position : Integrator  InitialCondition=init.FWR.P  ContinuousStateAttributes='position'
  velocity : Integrator  InitialCondition=init.FWR.V  ContinuousStateAttributes='velocity'
  "wdot -> w" : Integrator  InitialCondition=init.FWR.wbn
  FWR_r_plant_eci : Outport
  FWR_v_plant_eci : Outport  Port=2
  FWR_r_Sun2CS_plant_eci : Outport  Port=3
  FWR_r_MagField_plant_eci : Outport  Port=4
  FWR_quat_plant_body : Outport  Port=5
  FWR_rate_plant_body : Outport  Port=6
  wires:
  Add/1 -> FWR_r_Sun2CS_plant_eci/1, FWR_r_Sun2CS_plant_eci_scope/1
  ECI Position to LLA/1 -> Demux/1
  Sum1/1 -> Force2Accel/1
  Julian Date/1(Julian Date) -> Planetary Ephemeris/1
  Invert 3x3 Matrix/1 -> Product1/1
  Direction Cosine Matrix ECI to ECEF/1 -> Product/1, Invert 3x3 Matrix/1
  Demux/2 -> International Geomagnetic Reference Field 12/3
  Zonal Harmonic Gravity Model/1 -> Math Function/1
  FWR_F_app_eci/1 -> Sum1/2
  Product/1 -> Zonal Harmonic Gravity Model/1
  Demux/1 -> International Geomagnetic Reference Field 12/2
  Product1/1 -> Sum/2
  Sum/1 -> velocity/1
  Math Function/1 -> Product1/2
  Demux/3 -> International Geomagnetic Reference Field 12/1
  Force2Accel/1 -> Sum/1
  velocity/1 -> FWR_v_plant_eci/1, Atmospheric drag/1(velocity), position/1
  Planetary Ephemeris/1 -> Add/1
  International Geomagnetic Reference Field 12/1 -> FWR_r_MagField_plant_eci/1, FWR_r_MagField_plant_eci_scope/1
  DecimalYearIncrement/1(DecimalYear) -> International Geomagnetic Reference Field 12/4
  time_elapsed/1 -> Julian Date/1(deltaT), ECI Position to LLA/2, Direction Cosine Matrix ECI to ECEF/1, DecimalYearIncrement/1(clock_sec)
  FWR_h_rw_plant/1 -> Mux/1, "FWR_h_rw "/1, Sum4/2
  Cross/1(AxB) -> Sum3/3
  Sum4/1 -> Cross/2(B)
  Isc inverse/1 -> To Workspace2/1, "wdot -> w"/1
  "wdot -> w"/1 -> Inertia/1, Cross/1(A), To Workspace1/1, FWR_rate_plant_body/1, Quaternion Integration/1(w_Body), FWR_w_body/1
  Sum3/1 -> Isc inverse/1
  FWR_hb_rw_app/1 -> Mux/2, Sum3/2
  Mux/1 -> ?
  Inertia/1 -> Sum4/1
  Quaternion Integration/1(q_I_Body) -> Demux1/1, FWR_quat_plant_body/1
  Demux1/2 -> FWR_q/2
  Demux1/1 -> FWR_q/1
  Demux1/3 -> FWR_q/3
  Demux1/4 -> FWR_q/4
  Integrator1/1 -> Product4/2, norm/1(v), Product/2, Add/2, ECI Position to LLA/1, Position_FWR/1, FWR_r_plant_eci/1, Display1/1
  Earth's grav constant/1 -> Product2/1
  Product2/1 -> Gain/1
  Product3/1 -> Product2/2
  norm/1(|v|) -> Product3/3, Product3/2, Product3/1
  Integrator/1 -> Integrator1/1
  Product4/1 -> Integrator/1
  Gain/1 -> Product4/1

== system top_model_rw_desatTest/FWR_Sensor Model ==
  note: Gyroscope
  note: Magnetometer
  note: Sun Sensor
  note: GPS
  note: GPS
  FWR_r_plant_eci : Inport
  FWR_v_plant_eci : Inport  Port=2
  FWR_r_Sun2CS_plant_eci : Inport  Port=3
  FWR_r_MagField_plant_eci : Inport  Port=4
  FWR_quat_plant_body : Inport  Port=5
  FWR_rate_plant_body : Inport  Port=6
  time_elapsed : Inport  Port=7
  Direction Cosine Matrix ECI to ECEF : aerolibtransform2/Direction Cosine Matrix ECI to ECEF  red=IAU-2000/2006  year=init.year  month=October  day=20  hour=init.hour  min=init.min  sec=init.sec  deltaT=Sec  errorflag=Error  extraparamflag=off
      settings: AttributesFormatString=%<red>  SourceProductName=Aerospace Blockset  SourceProductBaseCode=AE
  Matrix Multiply{,1..3} (4 alike) : Product  Multiplication=Matrix(*)
  quat to DCM : Subsystem  mask(Direction Cosine Matrix){}
      mask help: Determines the 3x3 Direction Cosine Matrix (DCM) from a 4x1 quaternion orientation vector. The outputted DCM transforms vectors from inertial axes to body axes. This version corrects the fucked-up MATLAB one.
      mask Help:
      | <p>This block determines the 3x3 Direction Cosine Matrix (DCM) from a 4x1 quaternion orientation vector. The outputted DCM transforms vectors from inertial axes to body axes.  This version corrects the fucked-up MATLAB one</p>
      | 
      | <p>The block input and output contain more than one signal as described below.</p>
      | 
      | <p><H4>Block Vector Input - Quaternion</H4>
      | <ul>
      | <li>q0</li>
      | <li>q1</li>
      | <li>q2</li>
      | <li>q3</li>
      | </ul>
      | </p>
      | 
      | <p><H4>Block Matrix Output - Direction Cosine Matrix  </H4>
      |     <ul>
      |    </ul>
      |    </p>
      mask Display: disp('q to Q')
  FWR_r_sensor_ecef : Outport
  FWR_v_sensor_ecef : Outport  Port=2
  FWR_r_Sun2CS_sensor_body : Outport  Port=3
  FWR_r_MagField_sensor_body : Outport  Port=4
  FWR_rate_calc_body : Outport  Port=5
  wires:
  FWR_r_plant_eci/1 -> Matrix Multiply/2
  FWR_rate_plant_body/1 -> FWR_rate_calc_body/1
  FWR_quat_plant_body/1 -> quat to DCM/1(e0 e1 e2 e3)
  time_elapsed/1 -> Direction Cosine Matrix ECI to ECEF/1
  Direction Cosine Matrix ECI to ECEF/1 -> Matrix Multiply1/1, Matrix Multiply/1
  Matrix Multiply/1 -> FWR_r_sensor_ecef/1
  FWR_v_plant_eci/1 -> Matrix Multiply1/2
  Matrix Multiply1/1 -> FWR_v_sensor_ecef/1
  FWR_r_Sun2CS_plant_eci/1 -> Matrix Multiply3/2
  FWR_r_MagField_plant_eci/1 -> Matrix Multiply2/2
  Matrix Multiply3/1 -> FWR_r_Sun2CS_sensor_body/1
  Matrix Multiply2/1 -> FWR_r_MagField_sensor_body/1
  quat to DCM/1(DCM) -> Matrix Multiply3/1, Matrix Multiply2/1

== system top_model_rw_desatTest/GNC ==
  Follower Position : Inport
  Follower Velocity : Inport  Port=2
  Leader Position : Inport  Port=3
  Leader Velocity : Inport  Port=4
  Update Trigger : Inport  Port=5
  Follower Maneuver : Subsystem
  Follower Orbital Elements : Subsystem
  Leader Orbital Elements : Subsystem
  Mux : Mux  Inputs=6
  Mux1 : Mux  Inputs=6
  Params : Subsystem
  Target Orbit : MATLAB Function  TreatAsAtomicUnit=on
  pos_opt_eci : Outport
  Impulse_eci : Outport  Port=2
  ontime : Outport  Port=3
  wires:
  Follower Position/1 -> Follower Orbital Elements/1(r), Follower Maneuver/1(r_follower), Target Orbit/3(r_f)
  Follower Maneuver/2(pos_opt) -> pos_opt_eci/1
  [Imp_min] -> Follower Maneuver/7(Imp_min)
  Follower Maneuver/3(Impulse_eci) -> Impulse_eci/1
  Leader Orbital Elements/4(Ω) -> Mux/4
  Mux/1 -> Target Orbit/5(els_t)
  Follower Orbital Elements/6(θ) -> Mux1/6
  Follower Orbital Elements/2(e) -> Mux1/2
  Follower Orbital Elements/3(i) -> Mux1/3
  Update Trigger/1 -> Follower Maneuver/8(Update Trigger)
  Leader Velocity/1 -> Leader Orbital Elements/2(v), Target Orbit/2(v_t)
  [Imp_max] -> Follower Maneuver/6(Imp_max)
  Target Orbit/1(x_tgt) -> Follower Maneuver/4(x_tgt)
  [muE] -> Follower Maneuver/3(mu), Target Orbit/7(muE)
  [match_tol] -> Target Orbit/9(match_tol)
  [m_f] -> Follower Maneuver/5(m_follower)
  Follower Velocity/1 -> Follower Orbital Elements/2(v), Follower Maneuver/2(v_follower), Target Orbit/4(v_f)
  Follower Orbital Elements/1(a) -> Mux1/1
  Follower Orbital Elements/4(Ω) -> Mux1/4
  Leader Orbital Elements/5(ω) -> Mux/5
  Follower Maneuver/4(ontime) -> ontime/1
  Mux1/1 -> Target Orbit/6(els_f)
  Leader Orbital Elements/3(i) -> Mux/3
  Follower Orbital Elements/5(ω) -> Mux1/5
  Leader Orbital Elements/6(θ) -> Mux/6
  Leader Position/1 -> Leader Orbital Elements/1(r), Target Orbit/1(r_t)
  Leader Orbital Elements/1(a) -> Mux/1
  Leader Orbital Elements/2(e) -> Mux/2
  [K_F] -> Target Orbit/8(K_F)

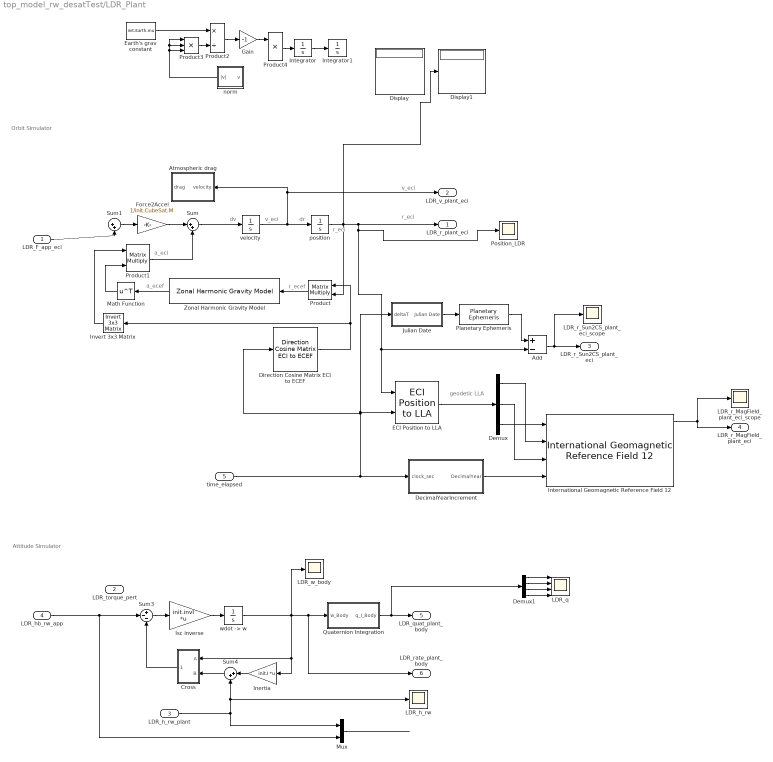
== system top_model_rw_desatTest/LDR_Plant ==
  note: a_ecef
  note: v_eci
  note: a_eci
  note: geodetic LLA
  note: r_ecef
  note: Orbit Simulator
  note: v_eci
  note: dv
  note: r_eci
  note: r_eci
  note: dr
  note: Attitude Simulator
  LDR_F_app_eci : Inport
  "LDR_torque_pert " : Inport  Port=2
  LDR_h_rw_plant : Inport  Port=3
  LDR_hb_rw_app : Inport  Port=4
  time_elapsed : Inport  Port=5
  Add : Sum  Inputs=+-
  Atmospheric drag : MATLAB Function  TreatAsAtomicUnit=on
  Cross : Subsystem
  DecimalYearIncrement : Subsystem
  Demux : Demux  Outputs=3
  Demux1 : Demux
  Direction Cosine Matrix ECI to ECEF : aerolibtransform2/Direction Cosine Matrix ECI to ECEF  red=IAU-2000/2006  year=init.year  month=October  day=20  hour=init.hour  min=init.min  sec=init.sec  deltaT=Sec  errorflag=Error  extraparamflag=off
      settings: AttributesFormatString=%<red>  SourceProductName=Aerospace Blockset  SourceProductBaseCode=AE
  Display : Display
  Display1 : Display
  ECI Position to LLA : aerolibtransform2/ECI Position to LLA  red=IAU-2000/2006  year=init.year  month=October  day=20  hour=init.hour  min=init.min  sec=init.sec  deltaT=Sec  errorflag=Error  extraparamflag=off  eunits=Metric (MKS)  earthmodel=WGS84  flat=1/298.257223563  eqradius=6378137
      settings: AttributesFormatString=%<red>  SourceProductName=Aerospace Blockset  SourceProductBaseCode=AE
  Earth's grav constant : Constant  Value=init.Earth.mu
  Force2Accel : Gain  Gain=1/init.CubeSat.M
  Gain : Gain  Gain=-1  SaturateOnIntegerOverflow=on  OutDataTypeStr=Inherit: Same as input  ParamDataTypeStr=Inherit: Same as input
  Inertia : Gain  Gain=init.I  Multiplication=Matrix(K*u)  SaturateOnIntegerOverflow=on  OutDataTypeStr=Inherit: Same as input  ParamDataTypeStr=Inherit: Same as input
  Integrator : Integrator  InitialCondition=init.LDR.V
  Integrator1 : Integrator  InitialCondition=init.LDR.P
  International Geomagnetic Reference Field 12 : aerolibgravity2/International Geomagnetic Reference Field 12  units=Metric (MKS)  time_in=on  month=January  day=1  year=2020  action=None  sv_out=off
      settings: SourceProductName=Aerospace Blockset  SourceProductBaseCode=AE
  Invert 3x3 Matrix : aerolibutil/Invert  3x3 Matrix
  Isc inverse : Gain  Gain=init.invI  Multiplication=Matrix(K*u)  SaturateOnIntegerOverflow=on  OutDataTypeStr=Inherit: Same as input  ParamDataTypeStr=Inherit: Same as input
  Julian Date : Subsystem
  "LDR_h_rw " : Scope
  LDR_q : Scope  NumInputPorts=4
  LDR_r_MagField_plant_eci_scope : Scope
  LDR_r_Sun2CS_plant_eci_scope : Scope
  LDR_w_body : Scope
  Math Function : Math  Operator=transpose  SaturateOnIntegerOverflow=on
  Mux : Mux  Inputs=2
  Planetary Ephemeris : aerolibcelestial/Planetary Ephemeris  kmflag=km,km/s  epochflag=Julian date  de=DE430  nCenter=Earth  nTarget=Sun  errorflag=Error  velflag=off
      settings: SourceProductName=Aerospace Blockset  SourceProductBaseCode=AE
  Position_LDR : Scope
  Product : Product  Multiplication=Matrix(*)
  Product1 : Product  Multiplication=Matrix(*)
  Product2 : Product  Inputs=*/  SaturateOnIntegerOverflow=on  OutDataTypeStr=Inherit: Same as first input
  Product3 : Product  Inputs=***  SaturateOnIntegerOverflow=on  OutDataTypeStr=Inherit: Same as first input
  Product4 : Product  Inputs=**  SaturateOnIntegerOverflow=on  OutDataTypeStr=Inherit: Same as first input
  Quaternion Integration : Subsystem
  Sum : Sum  Inputs=|++
  Sum1 : Sum  Inputs=|++
  Sum3 : Sum  Inputs=+--  SaturateOnIntegerOverflow=on  InputSameDT=on  OutDataTypeStr=Inherit: Same as first input
  Sum4 : Sum  Inputs=|++
  Zonal Harmonic Gravity Model : aerolibgravity2/Zonal Harmonic Gravity Model  units=Metric (MKS)  degree=4  action=Warning  ptype=Earth  R=6378136.3  GM=398600441500000  jvalue=[1.0826269e-03 -2.5323000e-06 -1.6204000e-06]
      settings: SourceProductName=Aerospace Blockset  SourceProductBaseCode=AE
  norm : Subsystem
  position : Integrator  InitialCondition=init.LDR.P  ContinuousStateAttributes='position'
  velocity : Integrator  InitialCondition=init.LDR.V  ContinuousStateAttributes='velocity'
  "wdot -> w" : Integrator  InitialCondition=init.LDR.wbn
  LDR_r_plant_eci : Outport
  LDR_v_plant_eci : Outport  Port=2
  LDR_r_Sun2CS_plant_eci : Outport  Port=3
  LDR_r_MagField_plant_eci : Outport  Port=4
  LDR_quat_plant_body : Outport  Port=5
  LDR_rate_plant_body : Outport  Port=6
  wires:
  Add/1 -> LDR_r_Sun2CS_plant_eci/1, LDR_r_Sun2CS_plant_eci_scope/1
  ECI Position to LLA/1 -> Demux/1
  Sum1/1 -> Force2Accel/1
  Julian Date/1(Julian Date) -> Planetary Ephemeris/1
  Invert 3x3 Matrix/1 -> Product1/1
  Direction Cosine Matrix ECI to ECEF/1 -> Product/1, Invert 3x3 Matrix/1
  Demux/2 -> International Geomagnetic Reference Field 12/3
  Zonal Harmonic Gravity Model/1 -> Math Function/1
  LDR_F_app_eci/1 -> Sum1/2
  Product/1 -> Zonal Harmonic Gravity Model/1
  Demux/1 -> International Geomagnetic Reference Field 12/2
  Product1/1 -> Sum/2
  Sum/1 -> velocity/1
  Math Function/1 -> Product1/2
  Demux/3 -> International Geomagnetic Reference Field 12/1
  Force2Accel/1 -> Sum/1
  velocity/1 -> LDR_v_plant_eci/1, Atmospheric drag/1(velocity), position/1
  Planetary Ephemeris/1 -> Add/1
  International Geomagnetic Reference Field 12/1 -> LDR_r_MagField_plant_eci/1, LDR_r_MagField_plant_eci_scope/1
  DecimalYearIncrement/1(DecimalYear) -> International Geomagnetic Reference Field 12/4
  time_elapsed/1 -> Julian Date/1(deltaT), ECI Position to LLA/2, Direction Cosine Matrix ECI to ECEF/1, DecimalYearIncrement/1(clock_sec)
  LDR_h_rw_plant/1 -> Mux/1, "LDR_h_rw "/1, Sum4/2
  Cross/1(AxB) -> Sum3/3
  Sum4/1 -> Cross/2(B)
  Isc inverse/1 -> "wdot -> w"/1
  "wdot -> w"/1 -> Inertia/1, Cross/1(A), LDR_rate_plant_body/1, Quaternion Integration/1(w_Body), LDR_w_body/1
  Sum3/1 -> Isc inverse/1
  LDR_hb_rw_app/1 -> Mux/2, Sum3/2
  Mux/1 -> ?
  Inertia/1 -> Sum4/1
  Quaternion Integration/1(q_I_Body) -> Demux1/1, LDR_quat_plant_body/1
  Demux1/2 -> LDR_q/2
  Demux1/1 -> LDR_q/1
  Demux1/3 -> LDR_q/3
  Demux1/4 -> LDR_q/4
  position/1 -> LDR_r_plant_eci/1, Position_LDR/1, Add/2, ECI Position to LLA/1, Product/2, Display1/1
  Earth's grav constant/1 -> Product2/1
  Product2/1 -> Gain/1
  Product3/1 -> Product2/2
  norm/1(|v|) -> Product3/3, Product3/2, Product3/1
  Integrator/1 -> Integrator1/1
  Product4/1 -> Integrator/1
  Gain/1 -> Product4/1

== system top_model_rw_desatTest/LDR_Sensor Model ==
  note: Gyroscope
  note: Magnetometer
  note: Sun Sensor
  note: GPS
  note: GPS
  LDR_r_plant_eci : Inport
  LDR_v_plant_eci : Inport  Port=2
  LDR_r_Sun2CS_plant_eci : Inport  Port=3
  LDR_r_MagField_plant_eci : Inport  Port=4
  LDR_quat_plant_body : Inport  Port=5
  LDR_rate_plant_body : Inport  Port=6
  time_elapsed : Inport  Port=7
  Direction Cosine Matrix ECI to ECEF : aerolibtransform2/Direction Cosine Matrix ECI to ECEF  red=IAU-2000/2006  year=init.year  month=October  day=20  hour=init.hour  min=init.min  sec=init.sec  deltaT=Sec  errorflag=Error  extraparamflag=off
      settings: AttributesFormatString=%<red>  SourceProductName=Aerospace Blockset  SourceProductBaseCode=AE
  Matrix Multiply{,1..3} (4 alike) : Product  Multiplication=Matrix(*)
  quat to DCM : Subsystem  mask(Direction Cosine Matrix){}
      mask help: Determines the 3x3 Direction Cosine Matrix (DCM) from a 4x1 quaternion orientation vector. The outputted DCM transforms vectors from inertial axes to body axes. This version corrects the fucked-up MATLAB one.
      mask Help:
      | <p>This block determines the 3x3 Direction Cosine Matrix (DCM) from a 4x1 quaternion orientation vector. The outputted DCM transforms vectors from inertial axes to body axes.  This version corrects the fucked-up MATLAB one</p>
      | 
      | <p>The block input and output contain more than one signal as described below.</p>
      | 
      | <p><H4>Block Vector Input - Quaternion</H4>
      | <ul>
      | <li>q0</li>
      | <li>q1</li>
      | <li>q2</li>
      | <li>q3</li>
      | </ul>
      | </p>
      | 
      | <p><H4>Block Matrix Output - Direction Cosine Matrix  </H4>
      |     <ul>
      |    </ul>
      |    </p>
      mask Display: disp('q to Q')
  LDR_r_sensor_ecef : Outport
  LDR_v_sensor_ecef : Outport  Port=2
  LDR_r_Sun2CS_sensor_body : Outport  Port=3
  LDR_r_MagField_sensor_body : Outport  Port=4
  LDR_rate_calc_body : Outport  Port=5
  wires:
  LDR_r_plant_eci/1 -> Matrix Multiply/2
  LDR_rate_plant_body/1 -> LDR_rate_calc_body/1
  LDR_quat_plant_body/1 -> quat to DCM/1(e0 e1 e2 e3)
  time_elapsed/1 -> Direction Cosine Matrix ECI to ECEF/1
  Direction Cosine Matrix ECI to ECEF/1 -> Matrix Multiply1/1, Matrix Multiply/1
  Matrix Multiply/1 -> LDR_r_sensor_ecef/1
  LDR_v_plant_eci/1 -> Matrix Multiply1/2
  Matrix Multiply1/1 -> LDR_v_sensor_ecef/1
  LDR_r_Sun2CS_plant_eci/1 -> Matrix Multiply3/2
  LDR_r_MagField_plant_eci/1 -> Matrix Multiply2/2
  Matrix Multiply3/1 -> LDR_r_Sun2CS_sensor_body/1
  Matrix Multiply2/1 -> LDR_r_MagField_sensor_body/1
  quat to DCM/1(DCM) -> Matrix Multiply3/1, Matrix Multiply2/1

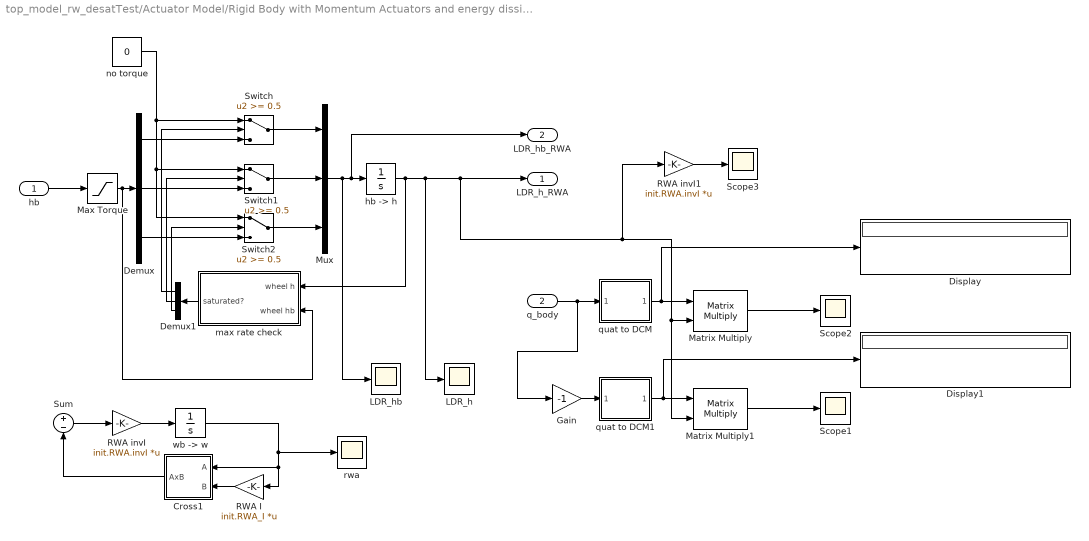
== system top_model_rw_desatTest/Actuator Model/Rigid Body with Momentum Actuators and energy dissipation ==
  hb : Inport
  q_body : Inport  Port=2
  Cross1 : Subsystem
  Demux : Demux  Outputs=3
  Demux1 : Demux  Outputs=3
  Display : Display
  Display1 : Display
  Gain : Gain  Gain=-1
  LDR_h : Scope
  LDR_hb : Scope
  Matrix Multiply : Product  Multiplication=Matrix(*)
  Matrix Multiply1 : Product  Multiplication=Matrix(*)
  Max Torque : Saturate  UpperLimit=init.hdmax  LowerLimit=-init.hdmax
  Mux : Mux  Inputs=3
  RWA I : Gain  Gain=init.RWA_I  Multiplication=Matrix(K*u)
  RWA invI : Gain  Gain=init.RWA.invI  Multiplication=Matrix(K*u)
  RWA invI1 : Gain  Gain=init.RWA.invI  Multiplication=Matrix(K*u)
  Scope1 : Scope
  Scope2 : Scope
  Scope3 : Scope
  Sum : Sum  Inputs=+|-
  Switch : Switch  Threshold=0.5  SaturateOnIntegerOverflow=on  InputSameDT=on
  Switch1 : Switch  Threshold=0.5  SaturateOnIntegerOverflow=on  InputSameDT=on
  Switch2 : Switch  Threshold=0.5  SaturateOnIntegerOverflow=on  InputSameDT=on
  "hb -> h" : Integrator  InitialCondition=init.LDR.h
  max rate check : Subsystem
  no torque : Constant  Value=0
  quat to DCM : Subsystem  mask(Direction Cosine Matrix){}
      mask help: Determines the 3x3 Direction Cosine Matrix (DCM) from a 4x1 quaternion orientation vector. The outputted DCM transforms vectors from inertial axes to body axes. This version corrects the fucked-up MATLAB one.
      mask Help:
      | <p>This block determines the 3x3 Direction Cosine Matrix (DCM) from a 4x1 quaternion orientation vector. The outputted DCM transforms vectors from inertial axes to body axes.  This version corrects the fucked-up MATLAB one</p>
      | 
      | <p>The block input and output contain more than one signal as described below.</p>
      | 
      | <p><H4>Block Vector Input - Quaternion</H4>
      | <ul>
      | <li>q0</li>
      | <li>q1</li>
      | <li>q2</li>
      | <li>q3</li>
      | </ul>
      | </p>
      | 
      | <p><H4>Block Matrix Output - Direction Cosine Matrix  </H4>
      |     <ul>
      |    </ul>
      |    </p>
      mask Display: disp('q to Q')
  quat to DCM1 : Subsystem  mask(Direction Cosine Matrix){}
      mask help: Determines the 3x3 Direction Cosine Matrix (DCM) from a 4x1 quaternion orientation vector. The outputted DCM transforms vectors from inertial axes to body axes. This version corrects the fucked-up MATLAB one.
      mask Help:
      | <p>This block determines the 3x3 Direction Cosine Matrix (DCM) from a 4x1 quaternion orientation vector. The outputted DCM transforms vectors from inertial axes to body axes.  This version corrects the fucked-up MATLAB one</p>
      | 
      | <p>The block input and output contain more than one signal as described below.</p>
      | 
      | <p><H4>Block Vector Input - Quaternion</H4>
      | <ul>
      | <li>q0</li>
      | <li>q1</li>
      | <li>q2</li>
      | <li>q3</li>
      | </ul>
      | </p>
      | 
      | <p><H4>Block Matrix Output - Direction Cosine Matrix  </H4>
      |     <ul>
      |    </ul>
      |    </p>
      mask Display: disp('q to Q')
  rwa : Scope
  "wb -> w" : Integrator  InitialCondition=[0;0;0]
  LDR_h_RWA : Outport
  LDR_hb_RWA : Outport  Port=2
  wires:
  hb/1 -> Max Torque/1
  Mux/1 -> LDR_hb_RWA/1, "hb -> h"/1, LDR_hb/1
  Max Torque/1 -> Demux/1, max rate check/2(wheel hb)
  max rate check/1(saturated?) -> Demux1/1
  Demux1/1 -> Switch/2
  Demux1/2 -> Switch1/2
  Demux1/3 -> Switch2/2
  no torque/1 -> Switch/1, Switch1/1, Switch2/1
  Demux/1 -> Switch/3
  Demux/2 -> Switch1/3
  Demux/3 -> Switch2/3
  Switch/1 -> Mux/1
  Switch1/1 -> Mux/2
  Switch2/1 -> Mux/3
  q_body/1 -> Gain/1, quat to DCM/1(e0 e1 e2 e3)
  quat to DCM/1(DCM) -> Display/1, Matrix Multiply/1
  Matrix Multiply/1 -> Scope2/1
  Matrix Multiply1/1 -> Scope1/1
  quat to DCM1/1(DCM) -> Display1/1, Matrix Multiply1/1
  "hb -> h"/1 -> max rate check/1(wheel h), RWA invI1/1, Matrix Multiply1/2, Matrix Multiply/2, LDR_h_RWA/1, LDR_h/1
  Gain/1 -> quat to DCM1/1(e0 e1 e2 e3)
  RWA I/1 -> Cross1/2(B)
  "wb -> w"/1 -> rwa/1, Cross1/1(A), RWA I/1
  Cross1/1(AxB) -> Sum/2
  Sum/1 -> RWA invI/1
  RWA invI/1 -> "wb -> w"/1
  RWA invI1/1 -> Scope3/1
  ? -> Sum/1

== system top_model_rw_desatTest/Actuator Model/torque_mt ==
  A : Inport
  B : Inport  Port=2
  Mux4 : Mux  Inputs=3
  Product{,1..5} (6 alike) : Product  SaturateOnIntegerOverflow=on  InputSameDT=on  OutDataTypeStr=Inherit: Same as first input
  Sum : Sum  Inputs=+-  SaturateOnIntegerOverflow=on  InputSameDT=on  OutDataTypeStr=Inherit: Same as first input
  Sum1 : Sum  Inputs=+-  SaturateOnIntegerOverflow=on  InputSameDT=on  OutDataTypeStr=Inherit: Same as first input
  Sum2 : Sum  Inputs=+-  SaturateOnIntegerOverflow=on  InputSameDT=on  OutDataTypeStr=Inherit: Same as first input
  demux2 : Demux  Outputs=3
  demux3 : Demux  Outputs=3
  AxB : Outport  InitialOutput=0
  wires:
  Mux4/1 -> AxB/1
  Sum2/1 -> Mux4/3
  Sum1/1 -> Mux4/2
  Sum/1 -> Mux4/1
  Product5/1 -> Sum2/2
  Product4/1 -> Sum2/1
  Product3/1 -> Sum1/2
  Product2/1 -> Sum1/1
  Product1/1 -> Sum/2
  Product/1 -> Sum/1
  demux3/1 -> Product5/2, Product2/2
  demux2/2 -> Product5/1, Product/1
  demux3/2 -> Product4/2, Product1/2
  demux2/1 -> Product4/1, Product3/1
  demux3/3 -> Product3/2, Product/2
  demux2/3 -> Product2/1, Product1/1
  B/1 -> demux3/1
  A/1 -> demux2/1
